simulink model "P3_12"  (R2024b)
settings: Solver=VariableStepAuto  StartTime=0.0  StopTime=30  RelTol=1e-3
settings Model: Creator=Rj Avro Biswas  LastModifiedBy=Rj Avro Biswas

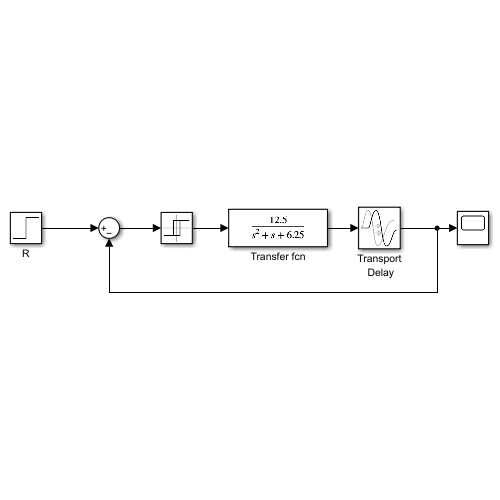
[thumbnail: Simulink's stored preview of the top-level diagram]
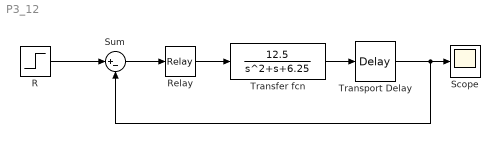
== system P3_12 ==
  R : Step  Before=5  After=10  SampleTime=0
  Relay : Relay  OnSwitchValue=1  OffSwitchValue=-1  OnOutputValue=2  OffOutputValue=-2
  Scope : Scope
  Sum : Sum  Inputs=|+-
  Transfer fcn : TransferFcn  Numerator=12.5  Denominator=[1 1 6.25]
  Transport Delay : TransportDelay  DelayTime=5
  wires:
  R/1 -> Sum/1
  Sum/1 -> Relay/1
  Relay/1 -> Transfer fcn/1
  Transfer fcn/1 -> Transport Delay/1
  Transport Delay/1 -> Sum/2, Scope/1
